simulink model "exampleOfWindPowerPlant"  (R2014b)
settings: Solver=FixedStepDiscrete  StartTime=0.0  StopTime=100000  FixedStep=1  RelTol=1e-3
undefined symbols (not defined in the file): DiSC_ToolboxOpal_V11, WindPowerPlant
(part 1 of 2)
settings Model: Creator=Rasmus  LastModifiedBy=seifu
settings DataIOCC: SignalLoggingSaveFormat=ModelDataLogs
settings DebuggingCC: MultiTaskDSMMsg=warning  MultiTaskCondExecSysMsg=none  StrictBusMsg=ErrorOnBusTreatedAsVector
settings RTWCC: IncludeERTFirstTime=on

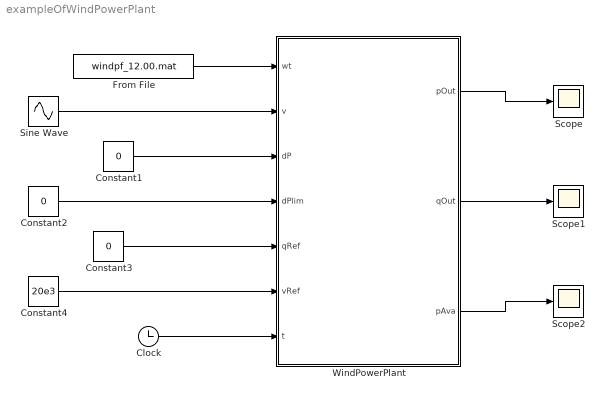
== system exampleOfWindPowerPlant ==
  Clock : Clock
  Constant1 : Constant  Value=0
  Constant2 : Constant  Value=0
  Constant3 : Constant  Value=0
  Constant4 : Constant  Value=20e3
  From File : FromFile  FileName=windpf_12.00.mat  SampleTime=0
  Scope : Scope
      settings: YMin=0  YMax=2e+07  MaxDataPoints=100000
  Scope1 : Scope
      settings: MaxDataPoints=100000
  Scope2 : Scope
      settings: SaveName=ScopeData2  MaxDataPoints=100000
  Sine Wave : Sin  Amplitude=2000  Bias=20e3  Frequency=0.00008  SampleTime=0
  WindPowerPlant : Subsystem  AncestorBlock=DiSC_ToolboxOpal_V11/WindPowerPlant  TreatAsAtomicUnit=on
      settings: RTWFcnNameOpts=Use subsystem name  RTWFileNameOpts=Use function name
  wires:
  From File/1 -> WindPowerPlant/1(wt)
  Sine Wave/1 -> WindPowerPlant/2(v)
  Constant1/1 -> WindPowerPlant/3(dP)
  Constant2/1 -> WindPowerPlant/4(dPlim)
  Constant3/1 -> WindPowerPlant/5(qRef)
  Constant4/1 -> WindPowerPlant/6(vRef)
  Clock/1 -> WindPowerPlant/7(t)
  WindPowerPlant/1(pOut) -> Scope/1
  WindPowerPlant/2(qOut) -> Scope1/1
  WindPowerPlant/3(pAva) -> Scope2/1

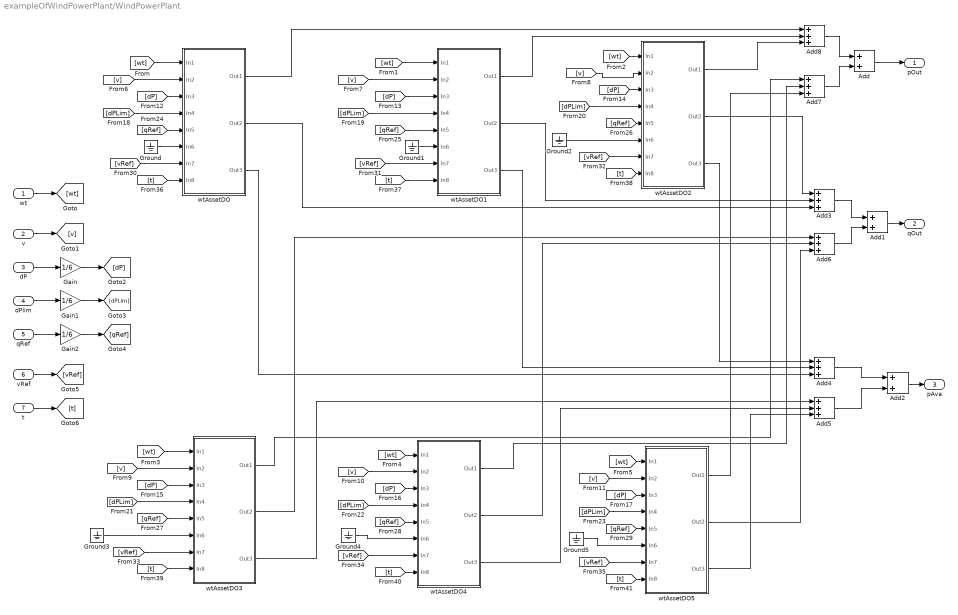
== system exampleOfWindPowerPlant/WindPowerPlant ==
  wt : Inport
  v : Inport  Port=2
  dP : Inport  Port=3
  dPlim : Inport  Port=4
  qRef : Inport  Port=5
  vRef : Inport  Port=6
  t : Inport  Port=7
  Add : Sum
  Add1 : Sum
  Add2 : Sum
  Add{3..8} (6 alike) : Sum  Inputs=+++
  Gain : Gain  Gain=1/6
  Gain1 : Gain  Gain=1/6
  Gain2 : Gain  Gain=1/6
  Ground{,1..5} (6 alike) : Ground
  wtAssetDO : Subsystem
      mask help:
      | %wtAssetS implements a simple P,Q controllable wind turbine system for Simulink.
      |     % This model works for Simulink and requires generatedWindFiles to
      |     % have been executed before running the simulink model
      |     %
      |     %   The wtAsset can be set to follow an active power reference, output
      |     %   maximum power available or curtail power. It can also, at the same
      |     %   time be set to follow a reactive power reference, output the
      |     %   minimum reactive power according to the power factor or try to keep
      |     %   a voltage reference in the coupling point by controlling reactive
      |     %   power output.
      |     %
      |     %   The model is partly based on the book
      |     %   "Optimal Control of Wind Energy Systems 2008".
      |     %
      |     %
      |     % Revision:
      |     % 23-05-2014, C. E. Sloth and R. Pedersen, Aalborg University. Notes:
      |     % 29-11-2014, R. Olsen/M. Kemal, Aalborg University (Simulink)
      |     % 20-06-2015, F. Iov/M. Kemal, Aalborg University (Simulink toolbox for OPAL)
      |             % Input:
      |             %   - w [m/s], is the wind speed.
      |             %   - v [PU], is the voltage at the connection point.
      |             %   - dP [PU], is the reference to active power change (curtailment).
      |             %   - dPlim [PU], is the reference to derated power (derate).
      |             %   - qRef [PU], is the reactive power reference.
      |             %   - vRef [PU], is the voltage reference.
      |             %
      |             % Output:
      |             %   - p [W], is active power outpur.
      |             %   - q [VAR], is reactive power output.
      |             %   - pAva [W], is the available active power
      mask Help:
      | %wtAssetS implements a simple P,Q controllable wind turbine system for Simulink.
      |     % This model works for Simulink and requires generatedWindFiles to
      |     % have been executed before running the simulink model
      |     %
      |     %   The wtAsset can be set to follow an active power reference, output
      |     %   maximum power available or curtail power. It can also, at the same
      |     %   time be set to follow a reactive power reference, output the
      |     %   minimum reactive power according to the power factor or try to keep
      |     %   a voltage reference in the coupling point by controlling reactive
      |     %   power output.
      |     %
      |     %   The model is partly based on the book
      |     %   "Optimal Control of Wind Energy Systems 2008".
      |     %
      |     %
      |     % Revision:
      |     % 23-05-2014, C. E. Sloth and R. Pedersen, Aalborg University. Notes:
      |     % 29-11-2014, R. Olsen/M. Kemal, Aalborg University (Simulink)
      |     % 20-06-2015, F. Iov/M. Kemal, Aalborg University (Simulink toolbox for OPAL)
      |             % Input:
      |             %   - w [m/s], is the wind speed.
      |             %   - v [PU], is the voltage at the connection point.
      |             %   - dP [PU], is the reference to active power change (curtailment).
      |             %   - dPlim [PU], is the reference to derated power (derate).
      |             %   - qRef [PU], is the reactive power reference.
      |             %   - vRef [PU], is the voltage reference.
      |             %
      |             % Output:
      |             %   - p [W], is active power outpur.
      |             %   - q [VAR], is reactive power output.
      |             %   - pAva [W], is the available active power
      mask Display:
      | image(imread( 'windTurbine.jpg'))
      | port_label( 'output',1, 'p')
      | port_label( 'output',2, 'q')
      | port_label( 'output',3, 'pAva')
      | 
      | 
      | port_label( 'input',1, 'wind')
      | port_label( 'input',2, 'vMeas')
      | port_label( 'input',3, 'dp')
      | port_label( 'input',4, 'dplim')
      | port_label( 'input',5, 'qRef')
      | port_label( 'input',6, 'qMode')
      | port_label( 'input',7, 'vRef')
      | port_label( 'input',8, 'time')
  wtAssetDO1 : Subsystem
      mask help:
      | %wtAssetS implements a simple P,Q controllable wind turbine system for Simulink.
      |     % This model works for Simulink and requires generatedWindFiles to
      |     % have been executed before running the simulink model
      |     %
      |     %   The wtAsset can be set to follow an active power reference, output
      |     %   maximum power available or curtail power. It can also, at the same
      |     %   time be set to follow a reactive power reference, output the
      |     %   minimum reactive power according to the power factor or try to keep
      |     %   a voltage reference in the coupling point by controlling reactive
      |     %   power output.
      |     %
      |     %   The model is partly based on the book
      |     %   "Optimal Control of Wind Energy Systems 2008".
      |     %
      |     %
      |     % Revision:
      |     % 23-05-2014, C. E. Sloth and R. Pedersen, Aalborg University. Notes:
      |     % 29-11-2014, R. Olsen/M. Kemal, Aalborg University (Simulink)
      |     % 20-06-2015, F. Iov/M. Kemal, Aalborg University (Simulink toolbox for OPAL)
      |             % Input:
      |             %   - w [m/s], is the wind speed.
      |             %   - v [PU], is the voltage at the connection point.
      |             %   - dP [PU], is the reference to active power change (curtailment).
      |             %   - dPlim [PU], is the reference to derated power (derate).
      |             %   - qRef [PU], is the reactive power reference.
      |             %   - vRef [PU], is the voltage reference.
      |             %
      |             % Output:
      |             %   - p [W], is active power outpur.
      |             %   - q [VAR], is reactive power output.
      |             %   - pAva [W], is the available active power
      mask Help:
      | %wtAssetS implements a simple P,Q controllable wind turbine system for Simulink.
      |     % This model works for Simulink and requires generatedWindFiles to
      |     % have been executed before running the simulink model
      |     %
      |     %   The wtAsset can be set to follow an active power reference, output
      |     %   maximum power available or curtail power. It can also, at the same
      |     %   time be set to follow a reactive power reference, output the
      |     %   minimum reactive power according to the power factor or try to keep
      |     %   a voltage reference in the coupling point by controlling reactive
      |     %   power output.
      |     %
      |     %   The model is partly based on the book
      |     %   "Optimal Control of Wind Energy Systems 2008".
      |     %
      |     %
      |     % Revision:
      |     % 23-05-2014, C. E. Sloth and R. Pedersen, Aalborg University. Notes:
      |     % 29-11-2014, R. Olsen/M. Kemal, Aalborg University (Simulink)
      |     % 20-06-2015, F. Iov/M. Kemal, Aalborg University (Simulink toolbox for OPAL)
      |             % Input:
      |             %   - w [m/s], is the wind speed.
      |             %   - v [PU], is the voltage at the connection point.
      |             %   - dP [PU], is the reference to active power change (curtailment).
      |             %   - dPlim [PU], is the reference to derated power (derate).
      |             %   - qRef [PU], is the reactive power reference.
      |             %   - vRef [PU], is the voltage reference.
      |             %
      |             % Output:
      |             %   - p [W], is active power outpur.
      |             %   - q [VAR], is reactive power output.
      |             %   - pAva [W], is the available active power
      mask Display:
      | image(imread( 'windTurbine.jpg'))
      | port_label( 'output',1, 'p')
      | port_label( 'output',2, 'q')
      | port_label( 'output',3, 'pAva')
      | 
      | 
      | port_label( 'input',1, 'wind')
      | port_label( 'input',2, 'vMeas')
      | port_label( 'input',3, 'dp')
      | port_label( 'input',4, 'dplim')
      | port_label( 'input',5, 'qRef')
      | port_label( 'input',6, 'qMode')
      | port_label( 'input',7, 'vRef')
      | port_label( 'input',8, 'time')
  wtAssetDO2 : Subsystem
      mask help:
      | %wtAssetS implements a simple P,Q controllable wind turbine system for Simulink.
      |     % This model works for Simulink and requires generatedWindFiles to
      |     % have been executed before running the simulink model
      |     %
      |     %   The wtAsset can be set to follow an active power reference, output
      |     %   maximum power available or curtail power. It can also, at the same
      |     %   time be set to follow a reactive power reference, output the
      |     %   minimum reactive power according to the power factor or try to keep
      |     %   a voltage reference in the coupling point by controlling reactive
      |     %   power output.
      |     %
      |     %   The model is partly based on the book
      |     %   "Optimal Control of Wind Energy Systems 2008".
      |     %
      |     %
      |     % Revision:
      |     % 23-05-2014, C. E. Sloth and R. Pedersen, Aalborg University. Notes:
      |     % 29-11-2014, R. Olsen/M. Kemal, Aalborg University (Simulink)
      |     % 20-06-2015, F. Iov/M. Kemal, Aalborg University (Simulink toolbox for OPAL)
      |             % Input:
      |             %   - w [m/s], is the wind speed.
      |             %   - v [PU], is the voltage at the connection point.
      |             %   - dP [PU], is the reference to active power change (curtailment).
      |             %   - dPlim [PU], is the reference to derated power (derate).
      |             %   - qRef [PU], is the reactive power reference.
      |             %   - vRef [PU], is the voltage reference.
      |             %
      |             % Output:
      |             %   - p [W], is active power outpur.
      |             %   - q [VAR], is reactive power output.
      |             %   - pAva [W], is the available active power
      mask Help:
      | %wtAssetS implements a simple P,Q controllable wind turbine system for Simulink.
      |     % This model works for Simulink and requires generatedWindFiles to
      |     % have been executed before running the simulink model
      |     %
      |     %   The wtAsset can be set to follow an active power reference, output
      |     %   maximum power available or curtail power. It can also, at the same
      |     %   time be set to follow a reactive power reference, output the
      |     %   minimum reactive power according to the power factor or try to keep
      |     %   a voltage reference in the coupling point by controlling reactive
      |     %   power output.
      |     %
      |     %   The model is partly based on the book
      |     %   "Optimal Control of Wind Energy Systems 2008".
      |     %
      |     %
      |     % Revision:
      |     % 23-05-2014, C. E. Sloth and R. Pedersen, Aalborg University. Notes:
      |     % 29-11-2014, R. Olsen/M. Kemal, Aalborg University (Simulink)
      |     % 20-06-2015, F. Iov/M. Kemal, Aalborg University (Simulink toolbox for OPAL)
      |             % Input:
      |             %   - w [m/s], is the wind speed.
      |             %   - v [PU], is the voltage at the connection point.
      |             %   - dP [PU], is the reference to active power change (curtailment).
      |             %   - dPlim [PU], is the reference to derated power (derate).
      |             %   - qRef [PU], is the reactive power reference.
      |             %   - vRef [PU], is the voltage reference.
      |             %
      |             % Output:
      |             %   - p [W], is active power outpur.
      |             %   - q [VAR], is reactive power output.
      |             %   - pAva [W], is the available active power
      mask Display:
      | image(imread( 'windTurbine.jpg'))
      | port_label( 'output',1, 'p')
      | port_label( 'output',2, 'q')
      | port_label( 'output',3, 'pAva')
      | 
      | 
      | port_label( 'input',1, 'wind')
      | port_label( 'input',2, 'vMeas')
      | port_label( 'input',3, 'dp')
      | port_label( 'input',4, 'dplim')
      | port_label( 'input',5, 'qRef')
      | port_label( 'input',6, 'qMode')
      | port_label( 'input',7, 'vRef')
      | port_label( 'input',8, 'time')
  wtAssetDO3 : Subsystem
      mask help:
      | %wtAssetS implements a simple P,Q controllable wind turbine system for Simulink.
      |     % This model works for Simulink and requires generatedWindFiles to
      |     % have been executed before running the simulink model
      |     %
      |     %   The wtAsset can be set to follow an active power reference, output
      |     %   maximum power available or curtail power. It can also, at the same
      |     %   time be set to follow a reactive power reference, output the
      |     %   minimum reactive power according to the power factor or try to keep
      |     %   a voltage reference in the coupling point by controlling reactive
      |     %   power output.
      |     %
      |     %   The model is partly based on the book
      |     %   "Optimal Control of Wind Energy Systems 2008".
      |     %
      |     %
      |     % Revision:
      |     % 23-05-2014, C. E. Sloth and R. Pedersen, Aalborg University. Notes:
      |     % 29-11-2014, R. Olsen/M. Kemal, Aalborg University (Simulink)
      |     % 20-06-2015, F. Iov/M. Kemal, Aalborg University (Simulink toolbox for OPAL)
      |             % Input:
      |             %   - w [m/s], is the wind speed.
      |             %   - v [PU], is the voltage at the connection point.
      |             %   - dP [PU], is the reference to active power change (curtailment).
      |             %   - dPlim [PU], is the reference to derated power (derate).
      |             %   - qRef [PU], is the reactive power reference.
      |             %   - vRef [PU], is the voltage reference.
      |             %
      |             % Output:
      |             %   - p [W], is active power outpur.
      |             %   - q [VAR], is reactive power output.
      |             %   - pAva [W], is the available active power
      mask Help:
      | %wtAssetS implements a simple P,Q controllable wind turbine system for Simulink.
      |     % This model works for Simulink and requires generatedWindFiles to
      |     % have been executed before running the simulink model
      |     %
      |     %   The wtAsset can be set to follow an active power reference, output
      |     %   maximum power available or curtail power. It can also, at the same
      |     %   time be set to follow a reactive power reference, output the
      |     %   minimum reactive power according to the power factor or try to keep
      |     %   a voltage reference in the coupling point by controlling reactive
      |     %   power output.
      |     %
      |     %   The model is partly based on the book
      |     %   "Optimal Control of Wind Energy Systems 2008".
      |     %
      |     %
      |     % Revision:
      |     % 23-05-2014, C. E. Sloth and R. Pedersen, Aalborg University. Notes:
      |     % 29-11-2014, R. Olsen/M. Kemal, Aalborg University (Simulink)
      |     % 20-06-2015, F. Iov/M. Kemal, Aalborg University (Simulink toolbox for OPAL)
      |             % Input:
      |             %   - w [m/s], is the wind speed.
      |             %   - v [PU], is the voltage at the connection point.
      |             %   - dP [PU], is the reference to active power change (curtailment).
      |             %   - dPlim [PU], is the reference to derated power (derate).
      |             %   - qRef [PU], is the reactive power reference.
      |             %   - vRef [PU], is the voltage reference.
      |             %
      |             % Output:
      |             %   - p [W], is active power outpur.
      |             %   - q [VAR], is reactive power output.
      |             %   - pAva [W], is the available active power
      mask Display:
      | image(imread( 'windTurbine.jpg'))
      | port_label( 'output',1, 'p')
      | port_label( 'output',2, 'q')
      | port_label( 'output',3, 'pAva')
      | 
      | 
      | port_label( 'input',1, 'wind')
      | port_label( 'input',2, 'vMeas')
      | port_label( 'input',3, 'dp')
      | port_label( 'input',4, 'dplim')
      | port_label( 'input',5, 'qRef')
      | port_label( 'input',6, 'qMode')
      | port_label( 'input',7, 'vRef')
      | port_label( 'input',8, 'time')
  wtAssetDO4 : Subsystem
      mask help:
      | %wtAssetS implements a simple P,Q controllable wind turbine system for Simulink.
      |     % This model works for Simulink and requires generatedWindFiles to
      |     % have been executed before running the simulink model
      |     %
      |     %   The wtAsset can be set to follow an active power reference, output
      |     %   maximum power available or curtail power. It can also, at the same
      |     %   time be set to follow a reactive power reference, output the
      |     %   minimum reactive power according to the power factor or try to keep
      |     %   a voltage reference in the coupling point by controlling reactive
      |     %   power output.
      |     %
      |     %   The model is partly based on the book
      |     %   "Optimal Control of Wind Energy Systems 2008".
      |     %
      |     %
      |     % Revision:
      |     % 23-05-2014, C. E. Sloth and R. Pedersen, Aalborg University. Notes:
      |     % 29-11-2014, R. Olsen/M. Kemal, Aalborg University (Simulink)
      |     % 20-06-2015, F. Iov/M. Kemal, Aalborg University (Simulink toolbox for OPAL)
      |             % Input:
      |             %   - w [m/s], is the wind speed.
      |             %   - v [PU], is the voltage at the connection point.
      |             %   - dP [PU], is the reference to active power change (curtailment).
      |             %   - dPlim [PU], is the reference to derated power (derate).
      |             %   - qRef [PU], is the reactive power reference.
      |             %   - vRef [PU], is the voltage reference.
      |             %
      |             % Output:
      |             %   - p [W], is active power outpur.
      |             %   - q [VAR], is reactive power output.
      |             %   - pAva [W], is the available active power
      mask Help:
      | %wtAssetS implements a simple P,Q controllable wind turbine system for Simulink.
      |     % This model works for Simulink and requires generatedWindFiles to
      |     % have been executed before running the simulink model
      |     %
      |     %   The wtAsset can be set to follow an active power reference, output
      |     %   maximum power available or curtail power. It can also, at the same
      |     %   time be set to follow a reactive power reference, output the
      |     %   minimum reactive power according to the power factor or try to keep
      |     %   a voltage reference in the coupling point by controlling reactive
      |     %   power output.
      |     %
      |     %   The model is partly based on the book
      |     %   "Optimal Control of Wind Energy Systems 2008".
      |     %
      |     %
      |     % Revision:
      |     % 23-05-2014, C. E. Sloth and R. Pedersen, Aalborg University. Notes:
      |     % 29-11-2014, R. Olsen/M. Kemal, Aalborg University (Simulink)
      |     % 20-06-2015, F. Iov/M. Kemal, Aalborg University (Simulink toolbox for OPAL)
      |             % Input:
      |             %   - w [m/s], is the wind speed.
      |             %   - v [PU], is the voltage at the connection point.
      |             %   - dP [PU], is the reference to active power change (curtailment).
      |             %   - dPlim [PU], is the reference to derated power (derate).
      |             %   - qRef [PU], is the reactive power reference.
      |             %   - vRef [PU], is the voltage reference.
      |             %
      |             % Output:
      |             %   - p [W], is active power outpur.
      |             %   - q [VAR], is reactive power output.
      |             %   - pAva [W], is the available active power
      mask Display:
      | image(imread( 'windTurbine.jpg'))
      | port_label( 'output',1, 'p')
      | port_label( 'output',2, 'q')
      | port_label( 'output',3, 'pAva')
      | 
      | 
      | port_label( 'input',1, 'wind')
      | port_label( 'input',2, 'vMeas')
      | port_label( 'input',3, 'dp')
      | port_label( 'input',4, 'dplim')
      | port_label( 'input',5, 'qRef')
      | port_label( 'input',6, 'qMode')
      | port_label( 'input',7, 'vRef')
      | port_label( 'input',8, 'time')
  wtAssetDO5 : Subsystem
      mask help:
      | %wtAssetS implements a simple P,Q controllable wind turbine system for Simulink.
      |     % This model works for Simulink and requires generatedWindFiles to
      |     % have been executed before running the simulink model
      |     %
      |     %   The wtAsset can be set to follow an active power reference, output
      |     %   maximum power available or curtail power. It can also, at the same
      |     %   time be set to follow a reactive power reference, output the
      |     %   minimum reactive power according to the power factor or try to keep
      |     %   a voltage reference in the coupling point by controlling reactive
      |     %   power output.
      |     %
      |     %   The model is partly based on the book
      |     %   "Optimal Control of Wind Energy Systems 2008".
      |     %
      |     %
      |     % Revision:
      |     % 23-05-2014, C. E. Sloth and R. Pedersen, Aalborg University. Notes:
      |     % 29-11-2014, R. Olsen/M. Kemal, Aalborg University (Simulink)
      |     % 20-06-2015, F. Iov/M. Kemal, Aalborg University (Simulink toolbox for OPAL)
      |             % Input:
      |             %   - w [m/s], is the wind speed.
      |             %   - v [PU], is the voltage at the connection point.
      |             %   - dP [PU], is the reference to active power change (curtailment).
      |             %   - dPlim [PU], is the reference to derated power (derate).
      |             %   - qRef [PU], is the reactive power reference.
      |             %   - vRef [PU], is the voltage reference.
      |             %
      |             % Output:
      |             %   - p [W], is active power outpur.
      |             %   - q [VAR], is reactive power output.
      |             %   - pAva [W], is the available active power
      mask Help:
      | %wtAssetS implements a simple P,Q controllable wind turbine system for Simulink.
      |     % This model works for Simulink and requires generatedWindFiles to
      |     % have been executed before running the simulink model
      |     %
      |     %   The wtAsset can be set to follow an active power reference, output
      |     %   maximum power available or curtail power. It can also, at the same
      |     %   time be set to follow a reactive power reference, output the
      |     %   minimum reactive power according to the power factor or try to keep
      |     %   a voltage reference in the coupling point by controlling reactive
      |     %   power output.
      |     %
      |     %   The model is partly based on the book
      |     %   "Optimal Control of Wind Energy Systems 2008".
      |     %
      |     %
      |     % Revision:
      |     % 23-05-2014, C. E. Sloth and R. Pedersen, Aalborg University. Notes:
      |     % 29-11-2014, R. Olsen/M. Kemal, Aalborg University (Simulink)
      |     % 20-06-2015, F. Iov/M. Kemal, Aalborg University (Simulink toolbox for OPAL)
      |             % Input:
      |             %   - w [m/s], is the wind speed.
      |             %   - v [PU], is the voltage at the connection point.
      |             %   - dP [PU], is the reference to active power change (curtailment).
      |             %   - dPlim [PU], is the reference to derated power (derate).
      |             %   - qRef [PU], is the reactive power reference.
      |             %   - vRef [PU], is the voltage reference.
      |             %
      |             % Output:
      |             %   - p [W], is active power outpur.
      |             %   - q [VAR], is reactive power output.
      |             %   - pAva [W], is the available active power
      mask Display:
      | image(imread( 'windTurbine.jpg'))
      | port_label( 'output',1, 'p')
      | port_label( 'output',2, 'q')
      | port_label( 'output',3, 'pAva')
      | 
      | 
      | port_label( 'input',1, 'wind')
      | port_label( 'input',2, 'vMeas')
      | port_label( 'input',3, 'dp')
      | port_label( 'input',4, 'dplim')
      | port_label( 'input',5, 'qRef')
      | port_label( 'input',6, 'qMode')
      | port_label( 'input',7, 'vRef')
      | port_label( 'input',8, 'time')
  pOut : Outport
  qOut : Outport  Port=2
  pAva : Outport  Port=3
  wires:
  Ground5/1 -> wtAssetDO5/6(In6)
  Ground4/1 -> wtAssetDO4/6(In6)
  Ground3/1 -> wtAssetDO3/6(In6)
  Ground2/1 -> wtAssetDO2/6(In6)
  Ground1/1 -> wtAssetDO1/6(In6)
  Ground/1 -> wtAssetDO/6(In6)
  [vRef] -> wtAssetDO5/7(In7)
  [t] -> wtAssetDO5/8(In8)
  [vRef] -> wtAssetDO/7(In7)
  Add/1 -> pOut/1
  Add7/1 -> Add/2
  Add8/1 -> Add/1
  wtAssetDO3/1(Out1) -> Add7/1
  wtAssetDO4/1(Out1) -> Add7/2
  wtAssetDO5/1(Out1) -> Add7/3
  Add1/1 -> qOut/1
  Add6/1 -> Add1/2
  Add3/1 -> Add1/1
  wtAssetDO3/2(Out2) -> Add6/1
  wtAssetDO4/2(Out2) -> Add6/2
  wtAssetDO5/2(Out2) -> Add6/3
  Add2/1 -> pAva/1
  Add5/1 -> Add2/2
  Add4/1 -> Add2/1
  wtAssetDO3/3(Out3) -> Add5/1
  wtAssetDO4/3(Out3) -> Add5/2
  wtAssetDO5/3(Out3) -> Add5/3
  wtAssetDO/3(Out3) -> Add4/3
  wtAssetDO1/3(Out3) -> Add4/2
  wtAssetDO2/3(Out3) -> Add4/1
  [t] -> wtAssetDO4/8(In8)
  [t] -> wtAssetDO3/8(In8)
  [t] -> wtAssetDO2/8(In8)
  [t] -> wtAssetDO1/8(In8)
  [t] -> wtAssetDO/8(In8)
  [vRef] -> wtAssetDO4/7(In7)
  [vRef] -> wtAssetDO3/7(In7)
  [vRef] -> wtAssetDO2/7(In7)
  [vRef] -> wtAssetDO1/7(In7)
  [qRef] -> wtAssetDO5/5(In5)
  [qRef] -> wtAssetDO4/5(In5)
  [qRef] -> wtAssetDO3/5(In5)
  [qRef] -> wtAssetDO2/5(In5)
  [qRef] -> wtAssetDO1/5(In5)
  [qRef] -> wtAssetDO/5(In5)
  [dPLim] -> wtAssetDO5/4(In4)
  [dPLim] -> wtAssetDO4/4(In4)
  [dPLim] -> wtAssetDO3/4(In4)
  [dPLim] -> wtAssetDO2/4(In4)
  [dPLim] -> wtAssetDO1/4(In4)
  [dPLim] -> wtAssetDO/4(In4)
  [dP] -> wtAssetDO5/3(In3)
  [dP] -> wtAssetDO4/3(In3)
  [dP] -> wtAssetDO3/3(In3)
  [dP] -> wtAssetDO2/3(In3)
  [dP] -> wtAssetDO1/3(In3)
  [dP] -> wtAssetDO/3(In3)
  [v] -> wtAssetDO5/2(In2)
  [v] -> wtAssetDO4/2(In2)
  [v] -> wtAssetDO3/2(In2)
  [v] -> wtAssetDO2/2(In2)
  [v] -> wtAssetDO1/2(In2)
  [v] -> wtAssetDO/2(In2)
  [wt] -> wtAssetDO5/1(In1)
  [wt] -> wtAssetDO4/1(In1)
  [wt] -> wtAssetDO3/1(In1)
  [wt] -> wtAssetDO2/1(In1)
  [wt] -> wtAssetDO1/1(In1)
  [wt] -> wtAssetDO/1(In1)
  wtAssetDO/2(Out2) -> Add3/3
  wtAssetDO1/2(Out2) -> Add3/2
  wtAssetDO2/2(Out2) -> Add3/1
  wtAssetDO/1(Out1) -> Add8/1
  wtAssetDO1/1(Out1) -> Add8/2
  wtAssetDO2/1(Out1) -> Add8/3
  t/1 -> [t]
  vRef/1 -> [vRef]
  Gain2/1 -> [qRef]
  Gain1/1 -> [dPLim]
  Gain/1 -> [dP]
  v/1 -> [v]
  wt/1 -> [wt]
  qRef/1 -> Gain2/1
  dPlim/1 -> Gain1/1
  dP/1 -> Gain/1

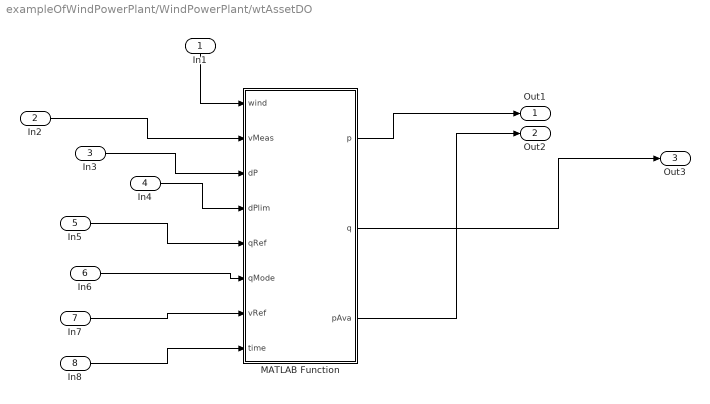
== system exampleOfWindPowerPlant/WindPowerPlant/wtAssetDO ==
  In1 : Inport
  In2 : Inport  Port=2
  In3 : Inport  Port=3
  In4 : Inport  Port=4
  In5 : Inport  Port=5
  In6 : Inport  Port=6
  In7 : Inport  Port=7
  In8 : Inport  Port=8
  MATLAB Function : MATLAB Function  TreatAsAtomicUnit=on
  Out1 : Outport
  Out2 : Outport  Port=2
  Out3 : Outport  Port=3
  wires:
  In8/1 -> MATLAB Function/8(time)
  In5/1 -> MATLAB Function/5(qRef)
  In6/1 -> MATLAB Function/6(qMode)
  In7/1 -> MATLAB Function/7(vRef)
  MATLAB Function/1(p) -> Out1/1
  In3/1 -> MATLAB Function/3(dP)
  In2/1 -> MATLAB Function/2(vMeas)
  MATLAB Function/2(q) -> Out3/1
  In4/1 -> MATLAB Function/4(dPlim)
  MATLAB Function/3(pAva) -> Out2/1
  In1/1 -> MATLAB Function/1(wind)

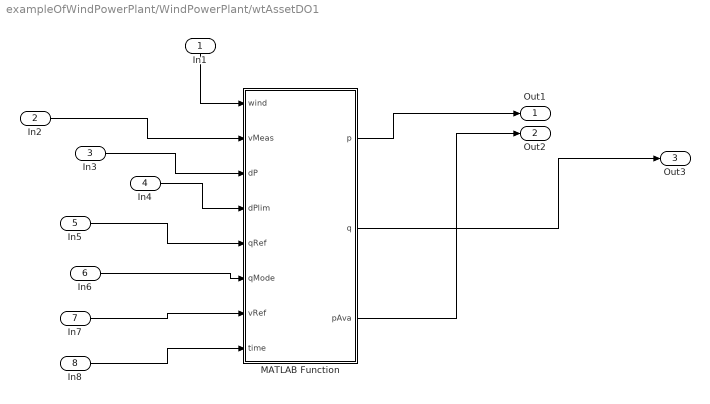
== system exampleOfWindPowerPlant/WindPowerPlant/wtAssetDO1 ==
  In1 : Inport
  In2 : Inport  Port=2
  In3 : Inport  Port=3
  In4 : Inport  Port=4
  In5 : Inport  Port=5
  In6 : Inport  Port=6
  In7 : Inport  Port=7
  In8 : Inport  Port=8
  MATLAB Function : MATLAB Function  TreatAsAtomicUnit=on
  Out1 : Outport
  Out2 : Outport  Port=2
  Out3 : Outport  Port=3
  wires:
  In8/1 -> MATLAB Function/8(time)
  In5/1 -> MATLAB Function/5(qRef)
  In6/1 -> MATLAB Function/6(qMode)
  In7/1 -> MATLAB Function/7(vRef)
  MATLAB Function/1(p) -> Out1/1
  In3/1 -> MATLAB Function/3(dP)
  In2/1 -> MATLAB Function/2(vMeas)
  MATLAB Function/2(q) -> Out3/1
  In4/1 -> MATLAB Function/4(dPlim)
  MATLAB Function/3(pAva) -> Out2/1
  In1/1 -> MATLAB Function/1(wind)

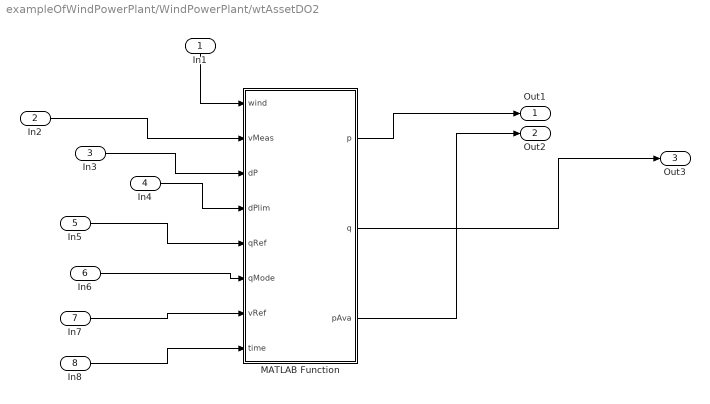
== system exampleOfWindPowerPlant/WindPowerPlant/wtAssetDO2 ==
  In1 : Inport
  In2 : Inport  Port=2
  In3 : Inport  Port=3
  In4 : Inport  Port=4
  In5 : Inport  Port=5
  In6 : Inport  Port=6
  In7 : Inport  Port=7
  In8 : Inport  Port=8
  MATLAB Function : MATLAB Function  TreatAsAtomicUnit=on
  Out1 : Outport
  Out2 : Outport  Port=2
  Out3 : Outport  Port=3
  wires:
  In8/1 -> MATLAB Function/8(time)
  In5/1 -> MATLAB Function/5(qRef)
  In6/1 -> MATLAB Function/6(qMode)
  In7/1 -> MATLAB Function/7(vRef)
  MATLAB Function/1(p) -> Out1/1
  In3/1 -> MATLAB Function/3(dP)
  In2/1 -> MATLAB Function/2(vMeas)
  MATLAB Function/2(q) -> Out3/1
  In4/1 -> MATLAB Function/4(dPlim)
  MATLAB Function/3(pAva) -> Out2/1
  In1/1 -> MATLAB Function/1(wind)

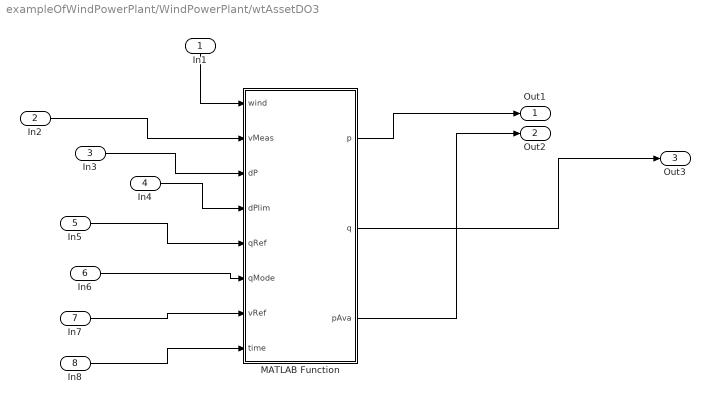
== system exampleOfWindPowerPlant/WindPowerPlant/wtAssetDO3 ==
  In1 : Inport
  In2 : Inport  Port=2
  In3 : Inport  Port=3
  In4 : Inport  Port=4
  In5 : Inport  Port=5
  In6 : Inport  Port=6
  In7 : Inport  Port=7
  In8 : Inport  Port=8
  MATLAB Function : MATLAB Function  TreatAsAtomicUnit=on
  Out1 : Outport
  Out2 : Outport  Port=2
  Out3 : Outport  Port=3
  wires:
  In8/1 -> MATLAB Function/8(time)
  In5/1 -> MATLAB Function/5(qRef)
  In6/1 -> MATLAB Function/6(qMode)
  In7/1 -> MATLAB Function/7(vRef)
  MATLAB Function/1(p) -> Out1/1
  In3/1 -> MATLAB Function/3(dP)
  In2/1 -> MATLAB Function/2(vMeas)
  MATLAB Function/2(q) -> Out3/1
  In4/1 -> MATLAB Function/4(dPlim)
  MATLAB Function/3(pAva) -> Out2/1
  In1/1 -> MATLAB Function/1(wind)

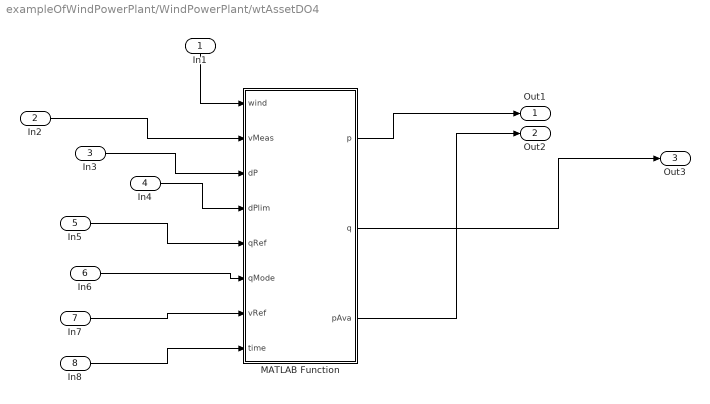
== system exampleOfWindPowerPlant/WindPowerPlant/wtAssetDO4 ==
  In1 : Inport
  In2 : Inport  Port=2
  In3 : Inport  Port=3
  In4 : Inport  Port=4
  In5 : Inport  Port=5
  In6 : Inport  Port=6
  In7 : Inport  Port=7
  In8 : Inport  Port=8
  MATLAB Function : MATLAB Function  TreatAsAtomicUnit=on
  Out1 : Outport
  Out2 : Outport  Port=2
  Out3 : Outport  Port=3
  wires:
  In8/1 -> MATLAB Function/8(time)
  In5/1 -> MATLAB Function/5(qRef)
  In6/1 -> MATLAB Function/6(qMode)
  In7/1 -> MATLAB Function/7(vRef)
  MATLAB Function/1(p) -> Out1/1
  In3/1 -> MATLAB Function/3(dP)
  In2/1 -> MATLAB Function/2(vMeas)
  MATLAB Function/2(q) -> Out3/1
  In4/1 -> MATLAB Function/4(dPlim)
  MATLAB Function/3(pAva) -> Out2/1
  In1/1 -> MATLAB Function/1(wind)

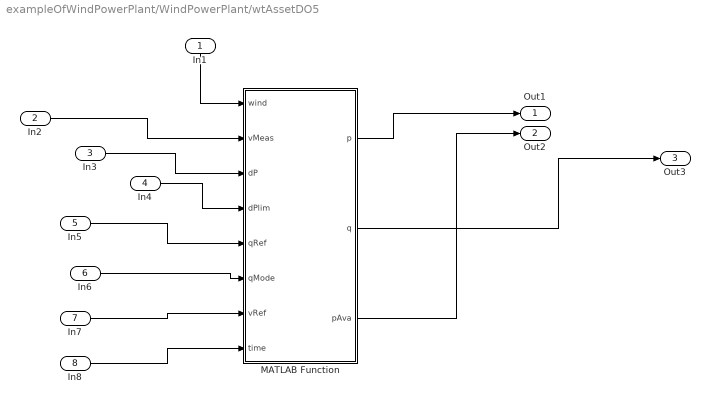
== system exampleOfWindPowerPlant/WindPowerPlant/wtAssetDO5 ==
  In1 : Inport
  In2 : Inport  Port=2
  In3 : Inport  Port=3
  In4 : Inport  Port=4
  In5 : Inport  Port=5
  In6 : Inport  Port=6
  In7 : Inport  Port=7
  In8 : Inport  Port=8
  MATLAB Function : MATLAB Function  TreatAsAtomicUnit=on
  Out1 : Outport
  Out2 : Outport  Port=2
  Out3 : Outport  Port=3
  wires:
  In8/1 -> MATLAB Function/8(time)
  In5/1 -> MATLAB Function/5(qRef)
  In6/1 -> MATLAB Function/6(qMode)
  In7/1 -> MATLAB Function/7(vRef)
  MATLAB Function/1(p) -> Out1/1
  In3/1 -> MATLAB Function/3(dP)
  In2/1 -> MATLAB Function/2(vMeas)
  MATLAB Function/2(q) -> Out3/1
  In4/1 -> MATLAB Function/4(dPlim)
  MATLAB Function/3(pAva) -> Out2/1
  In1/1 -> MATLAB Function/1(wind)

== matlab function exampleOfWindPowerPlant/WindPowerPlant/wtAssetDO/MATLAB Function ==
  data: p output; wind input; vMeas input; dP input; dPlim input; qRef input; qMode input; vRef input; time input; q output; pAva output
function [p,q,pAva] = wtAssetSDO(wind,vMeas,dP,dPlim,qRef,qMode,vRef, time)
%#codegen
    %wtAssetS implements a simple P,Q controllable wind turbine system for Simulink.
    % This model works for Simulink and requires generatedWindFiles to
    % have been executed before running the simulink model
    % 
    %   The wtAsset can be set to follow an active power reference, output
    %   maximum power available or curtail power. It can also, at the same
    %   time be set to follow a reactive power reference, output the
    %   minimum reactive power according to the power factor or try to keep
    %   a voltage reference in the coupling point by controlling reactive
    %   power output.
    %   
    %   The model is partly based on the book
    %   "Optimal Control of Wind Energy Systems 2008".
    %   
    %   
    % Revision:
    % 23-05-2014, C. E. Sloth and R. Pedersen, Aalborg University. Notes:
    % 29-11-2014, R. Olsen/M. Kemal, Aalborg University (Simulink)
         %Parameters
        param.vBase = 20e3;               % Voltage base [V].
        param.pRated = 100e3;               % Rated output power [W].
        param.sMax = 100e3;                 % Maximum apparent power [VA].
        param.wMin = 3;                   % Cut-in wind speed [m/s].
        param.wMax = 25;                  % Cut-out wind speed [m/s].
        param.wRated = 12;                % Rated wind speed [m/s].
        param.rfTau = 20;                 % Time constant of rotor filter [s].
        param.PF = 1;                     % Power factor [-].
        param.Ts = 60;                    % Sampling time [sec].  

     %variables 
     persistent var;
     if isempty(var)         
        var.p_c=0;                      %All used for caching in between sampling period
        var.q_c=0;
        var.pAva_c=0;
        var.t_c=0;
        var.pOld = 0;                   % [w]. Place holder for the rotor initia filter
        
        var.avgFilterTime = 10*60;      % [s]. Time that the filter should look back 
        var.avgFilterBuf = zeros(ceil(10*60/60),1);
        var.Qmode = 0;                  % [-]. Reactive power control mode
        var.kWT = 3e6/(12^3);           % [-]. Gain from w^3 to p
     end

            % Power conversion constant
            var.kWT = param.pRated/(param.wRated^3);    
            
            % Implement algorithm. 
            
            if (param.Ts>0)
               if (time>(var.t_c+param.Ts))
                   [p,q,pAva,varNew] = sampleWT(param,var,wind,vMeas,dP,dPlim,qRef,vRef);
                   varNew.p_c=p;
                   varNew.q_c=q;
                   varNew.pAva_c=pAva;
                   varNew.t_c=time;
                   varNew.Qmode = qMode;
                   var=varNew;
               end
               p=var.p_c;
               q=var.q_c;
               pAva=var.pAva_c;
            else
                [p,q,pAva,varNew] = sampleWT(param,var,wind,vMeas,dP,dPlim,qRef,vRef);
                var=varNew;
            end
            
        
            
%          [p,q,pAva,varNew] = sampleWT(obj,var,wind,vMeas,dP,dPlim,qRef,vRef);
         
         
end

== matlab function exampleOfWindPowerPlant/WindPowerPlant/wtAssetDO1/MATLAB Function ==
  data: p output; wind input; vMeas input; dP input; dPlim input; qRef input; qMode input; vRef input; time input; q output; pAva output
function [p,q,pAva] = wtAssetSDO(wind,vMeas,dP,dPlim,qRef,qMode,vRef, time)
%#codegen
    %wtAssetS implements a simple P,Q controllable wind turbine system for Simulink.
    % This model works for Simulink and requires generatedWindFiles to
    % have been executed before running the simulink model
    % 
    %   The wtAsset can be set to follow an active power reference, output
    %   maximum power available or curtail power. It can also, at the same
    %   time be set to follow a reactive power reference, output the
    %   minimum reactive power according to the power factor or try to keep
    %   a voltage reference in the coupling point by controlling reactive
    %   power output.
    %   
    %   The model is partly based on the book
    %   "Optimal Control of Wind Energy Systems 2008".
    %   
    %   
    % Revision:
    % 23-05-2014, C. E. Sloth and R. Pedersen, Aalborg University. Notes:
    % 29-11-2014, R. Olsen/M. Kemal, Aalborg University (Simulink)
         %Parameters
        param.vBase = 20e3;               % Voltage base [V].
        param.pRated = 100e3;               % Rated output power [W].
        param.sMax = 100e3;                 % Maximum apparent power [VA].
        param.wMin = 3;                   % Cut-in wind speed [m/s].
        param.wMax = 25;                  % Cut-out wind speed [m/s].
        param.wRated = 12;                % Rated wind speed [m/s].
        param.rfTau = 20;                 % Time constant of rotor filter [s].
        param.PF = 1;                     % Power factor [-].
        param.Ts = 60;                    % Sampling time [sec].  

     %variables 
     persistent var;
     if isempty(var)         
        var.p_c=0;                      %All used for caching in between sampling period
        var.q_c=0;
        var.pAva_c=0;
        var.t_c=0;
        var.pOld = 0;                   % [w]. Place holder for the rotor initia filter
        
        var.avgFilterTime = 10*60;      % [s]. Time that the filter should look back 
        var.avgFilterBuf = zeros(ceil(10*60/60),1);
        var.Qmode = 0;                  % [-]. Reactive power control mode
        var.kWT = 3e6/(12^3);           % [-]. Gain from w^3 to p
     end

            % Power conversion constant
            var.kWT = param.pRated/(param.wRated^3);    
            
            % Implement algorithm. 
            
            if (param.Ts>0)
               if (time>(var.t_c+param.Ts))
                   [p,q,pAva,varNew] = sampleWT(param,var,wind,vMeas,dP,dPlim,qRef,vRef);
                   varNew.p_c=p;
                   varNew.q_c=q;
                   varNew.pAva_c=pAva;
                   varNew.t_c=time;
                   varNew.Qmode = qMode;
                   var=varNew;
               end
               p=var.p_c;
               q=var.q_c;
               pAva=var.pAva_c;
            else
                [p,q,pAva,varNew] = sampleWT(param,var,wind,vMeas,dP,dPlim,qRef,vRef);
                var=varNew;
            end
            
        
            
%          [p,q,pAva,varNew] = sampleWT(obj,var,wind,vMeas,dP,dPlim,qRef,vRef);
         
         
end

== matlab function exampleOfWindPowerPlant/WindPowerPlant/wtAssetDO2/MATLAB Function ==
  data: p output; wind input; vMeas input; dP input; dPlim input; qRef input; qMode input; vRef input; time input; q output; pAva output
function [p,q,pAva] = wtAssetSDO(wind,vMeas,dP,dPlim,qRef,qMode,vRef, time)
%#codegen
    %wtAssetS implements a simple P,Q controllable wind turbine system for Simulink.
    % This model works for Simulink and requires generatedWindFiles to
    % have been executed before running the simulink model
    % 
    %   The wtAsset can be set to follow an active power reference, output
    %   maximum power available or curtail power. It can also, at the same
    %   time be set to follow a reactive power reference, output the
    %   minimum reactive power according to the power factor or try to keep
    %   a voltage reference in the coupling point by controlling reactive
    %   power output.
    %   
    %   The model is partly based on the book
    %   "Optimal Control of Wind Energy Systems 2008".
    %   
    %   
    % Revision:
    % 23-05-2014, C. E. Sloth and R. Pedersen, Aalborg University. Notes:
    % 29-11-2014, R. Olsen/M. Kemal, Aalborg University (Simulink)
         %Parameters
        param.vBase = 20e3;               % Voltage base [V].
        param.pRated = 100e3;               % Rated output power [W].
        param.sMax = 100e3;                 % Maximum apparent power [VA].
        param.wMin = 3;                   % Cut-in wind speed [m/s].
        param.wMax = 25;                  % Cut-out wind speed [m/s].
        param.wRated = 12;                % Rated wind speed [m/s].
        param.rfTau = 20;                 % Time constant of rotor filter [s].
        param.PF = 1;                     % Power factor [-].
        param.Ts = 60;                    % Sampling time [sec].  

     %variables 
     persistent var;
     if isempty(var)         
        var.p_c=0;                      %All used for caching in between sampling period
        var.q_c=0;
        var.pAva_c=0;
        var.t_c=0;
        var.pOld = 0;                   % [w]. Place holder for the rotor initia filter
        
        var.avgFilterTime = 10*60;      % [s]. Time that the filter should look back 
        var.avgFilterBuf = zeros(ceil(10*60/60),1);
        var.Qmode = 0;                  % [-]. Reactive power control mode
        var.kWT = 3e6/(12^3);           % [-]. Gain from w^3 to p
     end

            % Power conversion constant
            var.kWT = param.pRated/(param.wRated^3);    
            
            % Implement algorithm. 
            
            if (param.Ts>0)
               if (time>(var.t_c+param.Ts))
                   [p,q,pAva,varNew] = sampleWT(param,var,wind,vMeas,dP,dPlim,qRef,vRef);
                   varNew.p_c=p;
                   varNew.q_c=q;
                   varNew.pAva_c=pAva;
                   varNew.t_c=time;
                   varNew.Qmode = qMode;
                   var=varNew;
               end
               p=var.p_c;
               q=var.q_c;
               pAva=var.pAva_c;
            else
                [p,q,pAva,varNew] = sampleWT(param,var,wind,vMeas,dP,dPlim,qRef,vRef);
                var=varNew;
            end
            
        
            
%          [p,q,pAva,varNew] = sampleWT(obj,var,wind,vMeas,dP,dPlim,qRef,vRef);
         
         
end

== matlab function exampleOfWindPowerPlant/WindPowerPlant/wtAssetDO3/MATLAB Function ==
  data: p output; wind input; vMeas input; dP input; dPlim input; qRef input; qMode input; vRef input; time input; q output; pAva output
function [p,q,pAva] = wtAssetSDO(wind,vMeas,dP,dPlim,qRef,qMode,vRef, time)
%#codegen
    %wtAssetS implements a simple P,Q controllable wind turbine system for Simulink.
    % This model works for Simulink and requires generatedWindFiles to
    % have been executed before running the simulink model
    % 
    %   The wtAsset can be set to follow an active power reference, output
    %   maximum power available or curtail power. It can also, at the same
    %   time be set to follow a reactive power reference, output the
    %   minimum reactive power according to the power factor or try to keep
    %   a voltage reference in the coupling point by controlling reactive
    %   power output.
    %   
    %   The model is partly based on the book
    %   "Optimal Control of Wind Energy Systems 2008".
    %   
    %   
    % Revision:
    % 23-05-2014, C. E. Sloth and R. Pedersen, Aalborg University. Notes:
    % 29-11-2014, R. Olsen/M. Kemal, Aalborg University (Simulink)
         %Parameters
        param.vBase = 20e3;               % Voltage base [V].
        param.pRated = 100e3;               % Rated output power [W].
        param.sMax = 100e3;                 % Maximum apparent power [VA].
        param.wMin = 3;                   % Cut-in wind speed [m/s].
        param.wMax = 25;                  % Cut-out wind speed [m/s].
        param.wRated = 12;                % Rated wind speed [m/s].
        param.rfTau = 20;                 % Time constant of rotor filter [s].
        param.PF = 1;                     % Power factor [-].
        param.Ts = 60;                    % Sampling time [sec].  

     %variables 
     persistent var;
     if isempty(var)         
        var.p_c=0;                      %All used for caching in between sampling period
        var.q_c=0;
        var.pAva_c=0;
        var.t_c=0;
        var.pOld = 0;                   % [w]. Place holder for the rotor initia filter
        
        var.avgFilterTime = 10*60;      % [s]. Time that the filter should look back 
        var.avgFilterBuf = zeros(ceil(10*60/60),1);
        var.Qmode = 0;                  % [-]. Reactive power control mode
        var.kWT = 3e6/(12^3);           % [-]. Gain from w^3 to p
     end

            % Power conversion constant
            var.kWT = param.pRated/(param.wRated^3);    
            
            % Implement algorithm. 
            
            if (param.Ts>0)
               if (time>(var.t_c+param.Ts))
                   [p,q,pAva,varNew] = sampleWT(param,var,wind,vMeas,dP,dPlim,qRef,vRef);
                   varNew.p_c=p;
                   varNew.q_c=q;
                   varNew.pAva_c=pAva;
                   varNew.t_c=time;
                   varNew.Qmode = qMode;
                   var=varNew;
               end
               p=var.p_c;
               q=var.q_c;
               pAva=var.pAva_c;
            else
                [p,q,pAva,varNew] = sampleWT(param,var,wind,vMeas,dP,dPlim,qRef,vRef);
                var=varNew;
            end
            
        
            
%          [p,q,pAva,varNew] = sampleWT(obj,var,wind,vMeas,dP,dPlim,qRef,vRef);
         
         
end

== matlab function exampleOfWindPowerPlant/WindPowerPlant/wtAssetDO4/MATLAB Function ==
  data: p output; wind input; vMeas input; dP input; dPlim input; qRef input; qMode input; vRef input; time input; q output; pAva output
function [p,q,pAva] = wtAssetSDO(wind,vMeas,dP,dPlim,qRef,qMode,vRef, time)
%#codegen
    %wtAssetS implements a simple P,Q controllable wind turbine system for Simulink.
    % This model works for Simulink and requires generatedWindFiles to
    % have been executed before running the simulink model
    % 
    %   The wtAsset can be set to follow an active power reference, output
    %   maximum power available or curtail power. It can also, at the same
    %   time be set to follow a reactive power reference, output the
    %   minimum reactive power according to the power factor or try to keep
    %   a voltage reference in the coupling point by controlling reactive
    %   power output.
    %   
    %   The model is partly based on the book
    %   "Optimal Control of Wind Energy Systems 2008".
    %   
    %   
    % Revision:
    % 23-05-2014, C. E. Sloth and R. Pedersen, Aalborg University. Notes:
    % 29-11-2014, R. Olsen/M. Kemal, Aalborg University (Simulink)
         %Parameters
        param.vBase = 20e3;               % Voltage base [V].
        param.pRated = 100e3;               % Rated output power [W].
        param.sMax = 100e3;                 % Maximum apparent power [VA].
        param.wMin = 3;                   % Cut-in wind speed [m/s].
        param.wMax = 25;                  % Cut-out wind speed [m/s].
        param.wRated = 12;                % Rated wind speed [m/s].
        param.rfTau = 20;                 % Time constant of rotor filter [s].
        param.PF = 1;                     % Power factor [-].
        param.Ts = 60;                    % Sampling time [sec].  

     %variables 
     persistent var;
     if isempty(var)         
        var.p_c=0;                      %All used for caching in between sampling period
        var.q_c=0;
        var.pAva_c=0;
        var.t_c=0;
        var.pOld = 0;                   % [w]. Place holder for the rotor initia filter
        
        var.avgFilterTime = 10*60;      % [s]. Time that the filter should look back 
        var.avgFilterBuf = zeros(ceil(10*60/60),1);
        var.Qmode = 0;                  % [-]. Reactive power control mode
        var.kWT = 3e6/(12^3);           % [-]. Gain from w^3 to p
     end

            % Power conversion constant
            var.kWT = param.pRated/(param.wRated^3);    
            
            % Implement algorithm. 
            
            if (param.Ts>0)
               if (time>(var.t_c+param.Ts))
                   [p,q,pAva,varNew] = sampleWT(param,var,wind,vMeas,dP,dPlim,qRef,vRef);
                   varNew.p_c=p;
                   varNew.q_c=q;
                   varNew.pAva_c=pAva;
                   varNew.t_c=time;
                   varNew.Qmode = qMode;
                   var=varNew;
               end
               p=var.p_c;
               q=var.q_c;
               pAva=var.pAva_c;
            else
                [p,q,pAva,varNew] = sampleWT(param,var,wind,vMeas,dP,dPlim,qRef,vRef);
                var=varNew;
            end
            
        
            
%          [p,q,pAva,varNew] = sampleWT(obj,var,wind,vMeas,dP,dPlim,qRef,vRef);
         
         
end
